simulink model "Task_2_SSB"  (R2016a)
settings: Solver=VariableStepAuto  StartTime=0.0  StopTime=15  RelTol=1e-3
libraries: commanapbnd3 x2, dspsrcs4 x1
settings Model: Creator=92301  LastModifiedBy=92301

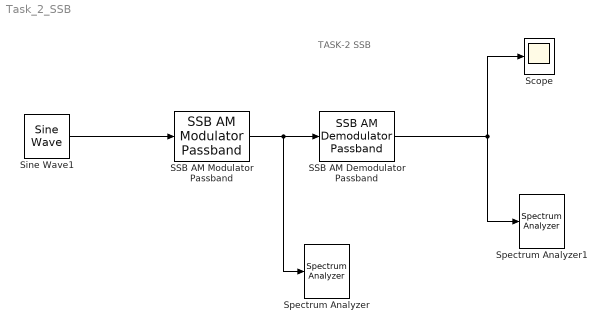
== system Task_2_SSB ==
  note: TASK-2 SSB
  SSB AM Demodulator Passband : commanapbnd3/SSB AM Demodulator Passband  Fc=2000  Ph=0  method=Butterworth  n=4  cf=300  Rp=0.1  Rs=50
  SSB AM Modulator Passband : commanapbnd3/SSB AM Modulator Passband  Fc=2000  Ph=0  Sd=Upper  Ho=100
  Scope : Scope
  "Sine Wave1 " : dspsrcs4/Sine Wave  Amplitude=5  Frequency=10  Phase=0  SampleMode=Discrete  OutComplex=Real  CompMethod=Trigonometric fcn  TableSize=Speed  SampleTime=1/1000  SamplesPerFrame=1  ResetState=Restart at time zero  OutputFrames=off  dataType=double  wordLen=16  udDataType=sfix(16)  fracBitsMode=Best precision  numFracBits=15  OutDataTypeStr=double  LastOutDataTypeStr=double
  "Spectrum Analyzer " : SpectrumAnalyzer
  "Spectrum Analyzer1 " : SpectrumAnalyzer
  wires:
  "Sine Wave1 "/1 -> SSB AM Modulator Passband/1
  SSB AM Modulator Passband/1 -> "Spectrum Analyzer "/1, SSB AM Demodulator Passband/1
  SSB AM Demodulator Passband/1 -> "Spectrum Analyzer1 "/1, Scope/1
